simulink model "lab_modulation_am"  (R2023a)
settings: Solver=VariableStepAuto  StartTime=0.0  StopTime=1  RelTol=1e-3
model workspace (MAT data in the model file):
  variance = Simulink.Parameter
  variance.Value = 0
  variance.Complexity = 'real'
  variance.Dimensions = [1 1]
  variance.DataType = 'auto'
values from neighbouring files (symbols this model uses):
  variance = 0.01    [lab_modulation_fm_saveas.m]    (also in lab_modulation_pm_saveas.m = 0)
libraries: dspfdesign x2
settings Model: Creator=andrey  LastModifiedBy=andrey
settings RTWCC: GPUComputeCapability=5.0

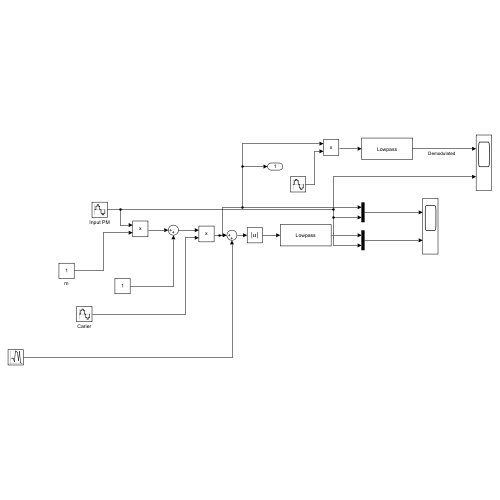
[thumbnail: Simulink's stored preview of the top-level diagram]
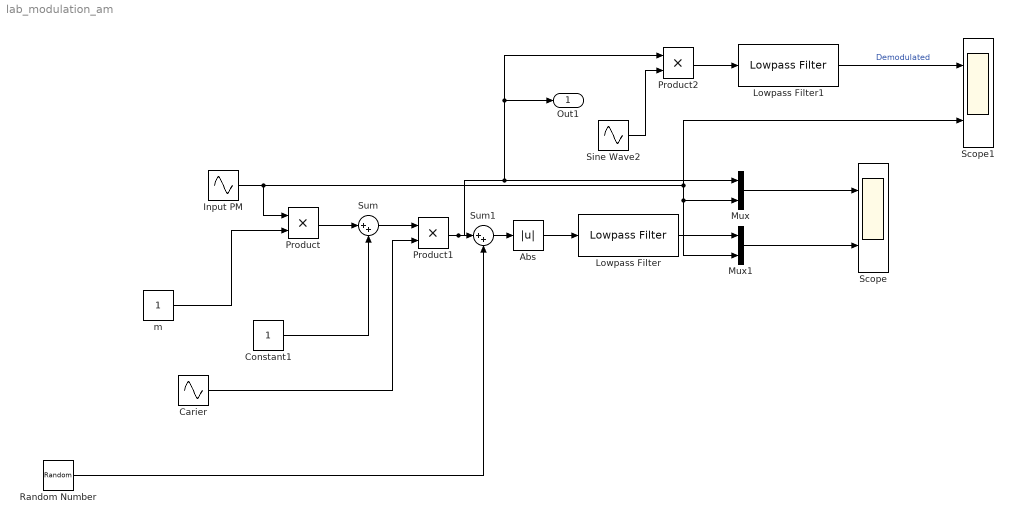
== system lab_modulation_am ==
  Abs : Abs  SaturateOnIntegerOverflow=off
  Carier : Sin  Frequency=100*2*pi  SampleTime=0.0001
  Constant1 : Constant
  Input PM : Sin  Frequency=2*2*pi  SampleTime=0.0001
  Lowpass Filter : dspfdesign/Lowpass Filter  FilterType=FIR  DesignForMinimumOrder=on  FilterOrder=50  PassbandFrequency=0.1  StopbandFrequency=100  PassbandRipple=0.1  StopbandAttenuation=80  SampleRate=44100  SimulateUsing=Interpreted execution  roundingMode=Floor  coeffsDataTypeStr=fixdt(1,16)
  Lowpass Filter1 : dspfdesign/Lowpass Filter  FilterType=FIR  DesignForMinimumOrder=on  FilterOrder=50  PassbandFrequency=10  StopbandFrequency=100  PassbandRipple=0.1  StopbandAttenuation=80  SampleRate=44100  SimulateUsing=Interpreted execution  roundingMode=Floor  coeffsDataTypeStr=fixdt(1,16)
  Mux : Mux  Inputs=2
  Mux1 : Mux  Inputs=2
  Product : Product
  Product1 : Product
  Product2 : Product
  Random Number : RandomNumber  Mean=0.5  Variance=variance  SampleTime=0.0001
  Scope : Scope  NumInputPorts=2
  Scope1 : Scope  NumInputPorts=2
  Sine Wave2 : Sin  Frequency=100*2*pi  SampleTime=0.0001
  Sum : Sum  Inputs=|++
  Sum1 : Sum  Inputs=|++
  m : Constant
  Out1 : Outport
  wires:
  m/1 -> Product/2
  Input PM/1 -> Mux/2, Mux1/2, Scope1/2, Product/1
  Product/1 -> Sum/1
  Constant1/1 -> Sum/2
  Sum/1 -> Product1/1
  Carier/1 -> Product1/2
  Product1/1 -> Mux/1, Product2/1, Out1/1, Sum1/1
  Abs/1 -> Lowpass Filter/1
  Lowpass Filter/1 -> Mux1/1
  Mux/1 -> Scope/1
  Mux1/1 -> Scope/2
  Sine Wave2/1 -> Product2/2
  Product2/1 -> Lowpass Filter1/1
  Lowpass Filter1/1 -> Scope1/1  "Demodulated"
  Sum1/1 -> Abs/1
  Random Number/1 -> Sum1/2
